simulink model "AM_Mod_coherent_tada_inc"  (R2015a)
settings: Solver=ode3  StartTime=0.0  StopTime=inf  FixedStep=1/22050  RelTol=1e-3
libraries: dspvision x1, dspsnks4 x1
settings Model: CovSFcnEnable=off  Creator=Ishraque  LastModifiedBy=cwang135
settings DebuggingCC: SolverPrmCheckMsg=warning

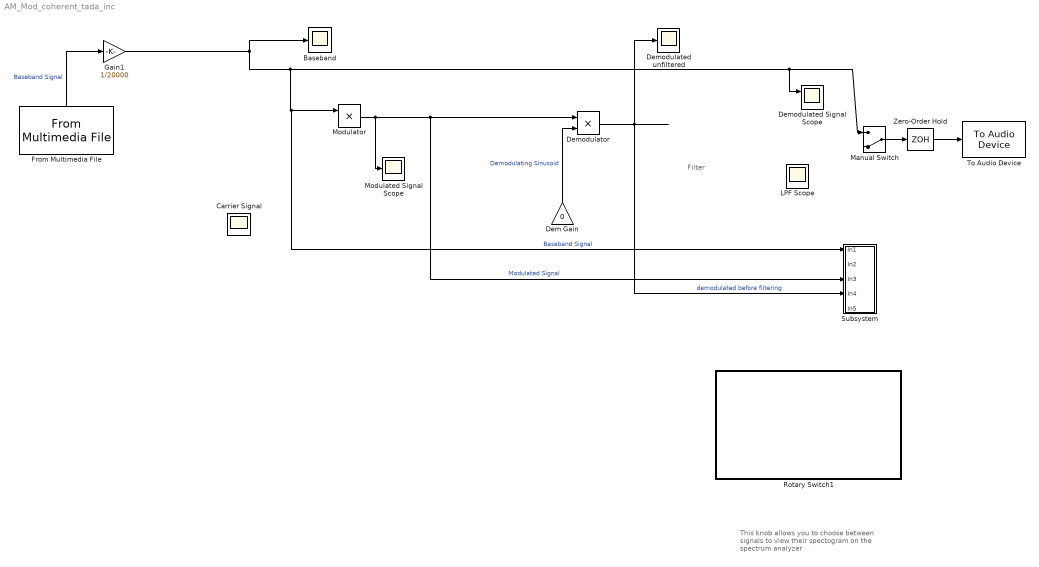
== system AM_Mod_coherent_tada_inc ==
  note: Filter
  note: This knob allows you to choose between
      | signals to view their spectogram on the
      | spectrum analyzer
  Baseband : Scope
      settings: TimeRange=10  TickLabels=on  MaxDataPoints=5000  SaveToWorkspace=off  YMin=-0.94969  YMax=1.03458  SampleTime=-1  DataFormat=Array
  "Carrier Signal " : Scope
      settings: TimeRange=50e-3  MaxDataPoints=5000  SaveToWorkspace=off  SaveName=ScopeData2  YMin=-1  YMax=1  SampleTime=-1  DataFormat=Array
  Dem Gain : Gain  Gain=0
  Demodulated Signal Scope : Scope  NumInputPorts=2
      settings: TimeRange=10  MaxDataPoints=5000  SaveToWorkspace=off  SaveName=ScopeData5  YMin=-1.15522~-0.96431  YMax=1.30882~1.04963  SampleTime=-1  DataFormat=Array
  Demodulated unfiltered : Scope
      settings: TimeRange=10  MaxDataPoints=5000  SaveToWorkspace=off  SaveName=ScopeData3  YMin=-4.89945  YMax=4.89851  SampleTime=-1  DataFormat=Array
  Demodulator : Product
  From Multimedia File : dspvision/From Multimedia File  inputFilename=tada.wav  loop=on  numPlays=inf  outputStreams=Audio only  videoDataType=single  audioDataType=int16  inheritSampleTime=on  userDefinedSampleTime=1/30  noAudioOutput=off  isIntensityVideo=off  fourcc=RGB  colorVideoFormat=One multidimensional signal  outputEOF=off  dataOrg=Column-major  audioFrameSize=1  computeAudioFrameSize=off  outSamplingMode=Sample based
  Gain1 : Gain  Gain=1/20000  OutDataTypeStr=double
  LPF Scope : Scope
      settings: TimeRange=10  MaxDataPoints=5000  SaveToWorkspace=off  SaveName=ScopeData4  YMin=-201.63677  YMax=204.52543  SampleTime=-1  DataFormat=Array
  Manual Switch : ManualSwitch  CurrentSetting=0
  Modulated Signal Scope : Scope
      settings: TimeRange=10  MaxDataPoints=5000  SaveToWorkspace=off  SaveName=ScopeData  YMin=-9.50868  YMax=9.51577  SampleTime=-1  DataFormat=Array
  Modulator : Product
  Rotary Switch1 : Subsystem  DialogController=hmiCreateDDGDialog  IsWebBlock=on  mask(MWDashboardBlock){webBlockId=534c7ef2-1674-4c23-9e54-a44f8668b583, webBlockType=discreteknob, ShowInLibBrowser=on, ShowInitialText=on, HMISrcModelName=AM_Mod_coherent_tada_inc_2015a}
      mask prompts: webBlockId "WebBlock Id"; webBlockType "WebBlock Type"; HMISrcModelName "Source Model"
      mask Help: helpview([docroot '/mapfiles/simulink.map'], 'hmi_rotary_switch')
      mask Display:
      | model = bdroot(gcb);
      | if strcmp(get_param(model,'BlockDiagramType'), 'library')
      |     image([(matlabroot) '/toolbox/simulink/hmi/icons/DiscreteKnob.png']);
      | end
  Subsystem : Subsystem
  To Audio Device : dspsnks4/To Audio Device  deviceName=Default  inheritSampleRate=on  sampleRate=44100  deviceDatatype=Determine from input data type  autoBufferSize=on  bufferSize=4096  queueDuration=1.0  defaultOutputChannelMapping=on  outputChannelMapping=1:2  outputNumUnderrunSamples=off
  Zero-Order Hold : ZeroOrderHold  SampleTime=1/22050
  wires:
  Modulator/1 -> Demodulator/1, Subsystem/3(In3), Modulated Signal Scope/1  "Modulated Signal"
  Demodulator/1 -> Subsystem/4(In4), Demodulated unfiltered/1  "demodulated before filtering"
  ? -> Demodulated Signal Scope/2, LPF Scope/1, Manual Switch/2, Subsystem/5(In5)  "Demodulated Filtered Signal"
  ? -> Dem Gain/1, Subsystem/2(In2), Modulator/2, "Carrier Signal "/1  "Carrier Signal"
  Dem Gain/1 -> Demodulator/2  "Demodulating Sinusoid"
  Gain1/1 -> Subsystem/1(In1), Modulator/1, Demodulated Signal Scope/1, Manual Switch/1, Baseband/1  "Baseband Signal"
  From Multimedia File/1 -> Gain1/1  "Baseband Signal"
  Manual Switch/1 -> Zero-Order Hold/1
  Zero-Order Hold/1 -> To Audio Device/1

== system AM_Mod_coherent_tada_inc/Rotary Switch1 ==

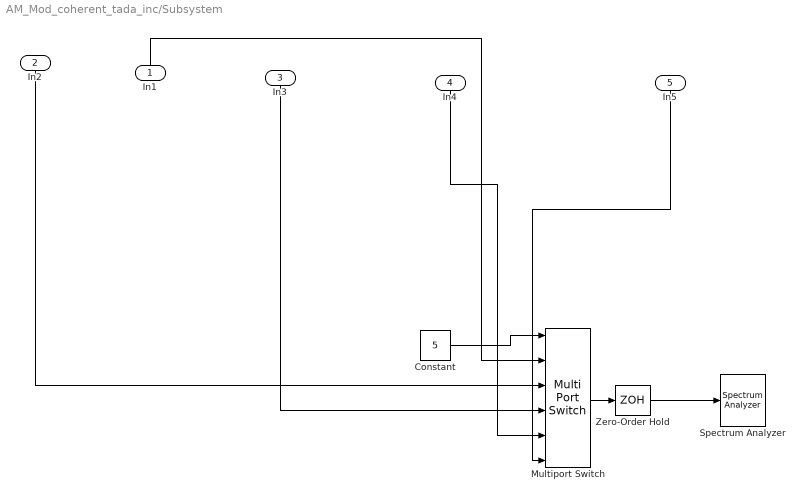
== system AM_Mod_coherent_tada_inc/Subsystem ==
  In1 : Inport
  In2 : Inport  Port=2
  In3 : Inport  Port=3
  In4 : Inport  Port=4
  In5 : Inport  Port=5
  Constant : Constant  Value=5
  Multiport Switch : MultiPortSwitch  Inputs=5
  Spectrum Analyzer : SpectrumAnalyzer
  Zero-Order Hold : ZeroOrderHold  SampleTime=1/22050
  wires:
  Zero-Order Hold/1 -> Spectrum Analyzer/1
  Multiport Switch/1 -> Zero-Order Hold/1
  Constant/1 -> Multiport Switch/1
  In1/1 -> Multiport Switch/2
  In2/1 -> Multiport Switch/3
  In4/1 -> Multiport Switch/5
  In5/1 -> Multiport Switch/6
  In3/1 -> Multiport Switch/4
